simulink model "sampleModel1861"  (R2023a)
settings: Solver=VariableStepAuto  StartTime=0.0  StopTime=10.0  RelTol=1e-3
libraries: simulink x6, hdlsllib x5
settings Model: Creator=user1  LastModifiedBy=user1

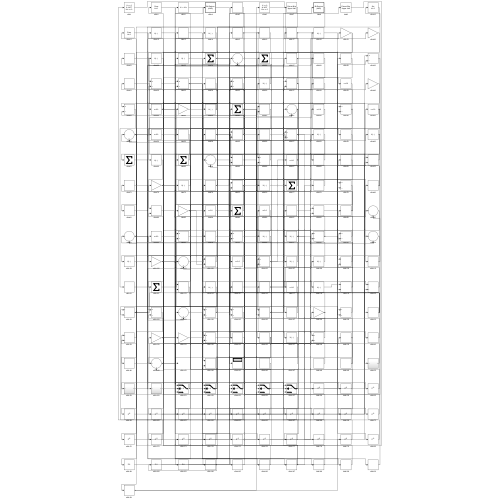
[thumbnail: Simulink's stored preview of the top-level diagram]
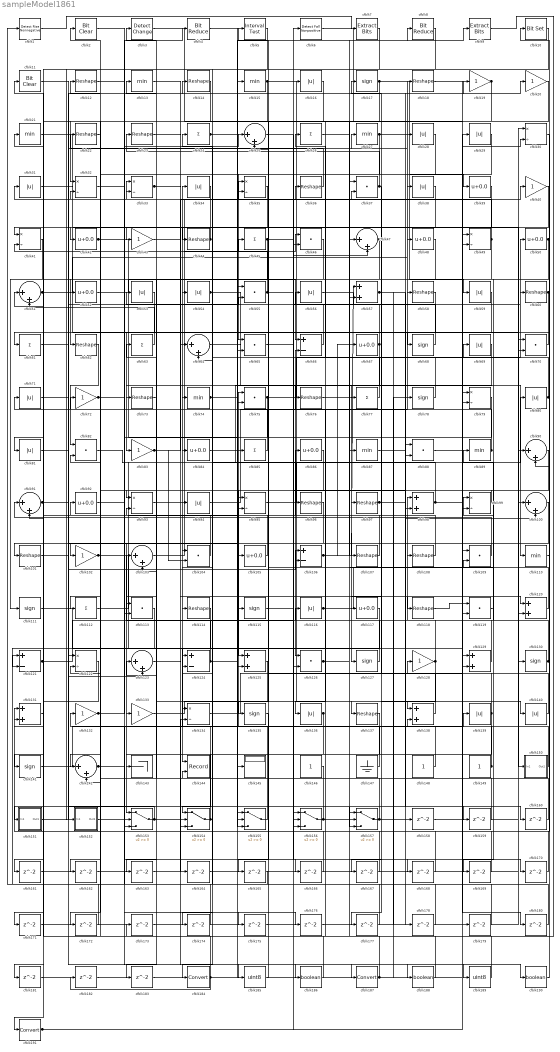
== system sampleModel1861 ==
  cfblk1 : hdlsllib/Logic and Bit Operations/Detect Rise Nonnegative  vinit=0  OutDataTypeStr=boolean
  cfblk10 : simulink/Logic and Bit Operations/Bit Set  iBit=0
      settings: LibrarySourceBlock=|
      | hdlsllib/Logic and Bit
      | Operations/Bit Set
  cfblk{25,47,51,64,90..91,100,103,123,142} (10 alike) : Sum  Inputs=|++
  cfblk{12,14,18,22..23,36,44,58,60,62,73,76,96..97,101,107..108,114,118,137} (20 alike) : Reshape
  cfblk{19..20,40,43,72,83,102,128,132..133} (10 alike) : Gain
  cfblk{37,46,55,65,70,75,82,88,104,109,113,119,126} (13 alike) : DotProduct  OutDataTypeStr=Inherit: Inherit via internal rule
  cfblk{39,42,48,50,52,67,84,86,92,105,117} (11 alike) : Bias  Bias=0.0  SaturateOnIntegerOverflow=off
  cfblk{66,106,121,124} (4 alike) : Sum  Inputs=+-
  cfblk11 : simulink/Logic and Bit Operations/Bit Clear  iBit=0
      settings: LibrarySourceBlock=|
      | hdlsllib/Logic and Bit
      | Operations/Bit Clear
  cfblk{13,15,21,27,74,87,89,110} (8 alike) : MinMax
  cfblk{17,68,78,111,115,127,130,135,141} (9 alike) : Signum
  cfblk{24,26,45,61,63,77,85,112} (8 alike) : Sum  Inputs=+
  cfblk{16,28..29,31,34,38,53..54,56,59,69,71,80..81,94,116,136,139..140} (19 alike) : Abs  SaturateOnIntegerOverflow=off
  cfblk{57,98,120,125,129,131,138} (7 alike) : Sum
  cfblk{30,32..33,35,41,49,79,93,95,99,122,134} (12 alike) : Product  Inputs=*/  RndMeth=Zero  SaturateOnIntegerOverflow=on
  cfblk143 : Terminator
  cfblk144 : Record  FileSettingsInternal="{\"entries\":[{\"content\":{\"excelSettings\":{\"content\":{},\"type\":\"Streamout.ExcelSettings\"}},\"type\":\"Streamout.FileSettingStorage\",\"uuid\":\"\"}],\"packageUris\":[\"http:\\/\\/schema.mathworks.com\\/mf0\\/streamout_blocks\\/R2020a\"],\"version\":\"1.0\"}"  Layout=[1 1]  SignalsInternal="{\"entries\":[{\"content\":{\"signals\":[{\"content\":{\"blockPath\":[],\"dimensions\":[1],\"domain\":\"\",\"lineColor\":\"#a2142f\",\"plots\":[1],\"port\":1,\"signalID\":4612,\"signalName\":\"XY Graph:1\"},\"type\":\"RecordBlkView.Signal\",\"uuid\":\"\"},{\"content\":{\"blockPath\":[],\"dimensions\":[1],\"domain\":\"\",\"lineColor\":\"#139fff\",\"plots\":[1],\"port\":2,\"signalID\":4615,\"signalName\":\"XY Graph:2\"},\"type\":\"RecordBlkView.Signal\",\"uuid\":\"\"}]},\"type\":\"RecordBlkView.InputSignals\",\"uuid\":\"\"}],\"packageUris\":[\"http:\\/\\/schema.mathworks.com\\/mf0\\/streamout_blocks\\/R2020a\"],\"version\":\"1.0\"}"  VisualizationBindings="{\"xyplotplugin\":{\"info\":[{\"series\":[{\"bindingParametersList\":[{\"parameter\":\"X-Axis\",\"signalID\":4612,\"signalName\":\"XY Graph:1\"},{\"parameter\":\"Y-Axis\",\"signalID\":4615,\"signalName\":\"XY Graph:2\"}],\"seriesID\":8507}],\"subplotID\":1}]}}"  CompatibilityTag=XY  st=-1
  cfblk145 : Display
  cfblk146 : Constant  SampleTime=-1
  cfblk147 : Ground
  cfblk148 : Constant  SampleTime=-1
  cfblk149 : Constant  SampleTime=-1
  cfblk150 : Subsystem
      settings: LibrarySourceBlock=|
      | hdlsllib/Ports &
      | Subsystems/Subsystem
  cfblk151 : Subsystem
      settings: LibrarySourceBlock=|
      | hdlsllib/Ports &
      | Subsystems/Subsystem
  cfblk152 : Subsystem
      settings: LibrarySourceBlock=|
      | hdlsllib/Ports &
      | Subsystems/Subsystem
  cfblk{153..157} (5 alike) : Switch  SaturateOnIntegerOverflow=off  InputSameDT=off
  cfblk{158..183} (26 alike) : Delay  SampleTime=1
  cfblk184 : DataTypeConversion  SaturateOnIntegerOverflow=off  RndMeth=Floor
  cfblk185 : DataTypeConversion  OutDataTypeStr=uint8  SaturateOnIntegerOverflow=off  RndMeth=Floor
  cfblk186 : DataTypeConversion  OutDataTypeStr=boolean  SaturateOnIntegerOverflow=off  RndMeth=Floor
  cfblk187 : DataTypeConversion  SaturateOnIntegerOverflow=off  RndMeth=Floor
  cfblk188 : DataTypeConversion  OutDataTypeStr=boolean  SaturateOnIntegerOverflow=off  RndMeth=Floor
  cfblk189 : DataTypeConversion  OutDataTypeStr=uint8  SaturateOnIntegerOverflow=off  RndMeth=Floor
  cfblk190 : DataTypeConversion  OutDataTypeStr=boolean  SaturateOnIntegerOverflow=off  RndMeth=Floor
  cfblk191 : DataTypeConversion  SaturateOnIntegerOverflow=off  RndMeth=Floor
  cfblk2 : simulink/Logic and Bit Operations/Bit Clear  iBit=0
      settings: LibrarySourceBlock=|
      | hdlsllib/Logic and Bit
      | Operations/Bit Clear
  cfblk3 : simulink/Logic and Bit Operations/Detect Change  vinit=0  OutDataTypeStr=boolean
      settings: LibrarySourceBlock=|
      | hdlsllib/Logic and Bit
      | Operations/Detect
      | Change
  cfblk4 : hdlsllib/Logic and Bit Operations/Bit Reduce  mode=AND
  cfblk5 : hdlsllib/Logic and Bit Operations/Interval Test  IntervalClosedRight=on  uplimit=0.5  IntervalClosedLeft=on  lowlimit=-0.5  OutDataTypeStr=boolean
  cfblk6 : hdlsllib/Logic and Bit Operations/Detect Fall Nonpositive  vinit=0  OutDataTypeStr=boolean
  cfblk7 : simulink/Logic and Bit Operations/Extract Bits  bitsToExtract=Upper half  numBits=8  bitIdxRange=[0 7]  outScalingMode=Preserve fixed-point scaling
      settings: LibrarySourceBlock=|
      | hdlsllib/Logic and Bit
      | Operations/Extract Bits
  cfblk8 : hdlsllib/Logic and Bit Operations/Bit Reduce  mode=AND
  cfblk9 : simulink/Logic and Bit Operations/Extract Bits  bitsToExtract=Upper half  numBits=8  bitIdxRange=[0 7]  outScalingMode=Preserve fixed-point scaling
      settings: LibrarySourceBlock=|
      | hdlsllib/Logic and Bit
      | Operations/Extract Bits
  wires:
  cfblk108/1 -> cfblk75/1
  cfblk155/1 -> cfblk132/1
  cfblk150/1(Out1) -> cfblk75/2
  cfblk53/1 -> cfblk83/1
  cfblk82/1 -> cfblk110/1
  cfblk8/1 -> cfblk152/1(In1)
  cfblk96/1 -> cfblk153/1
  cfblk15/1 -> cfblk137/1, cfblk142/2
  cfblk138/1 -> cfblk128/1
  cfblk109/1 -> cfblk91/1
  cfblk118/1 -> cfblk119/1
  cfblk133/1 -> cfblk138/1
  cfblk113/1 -> cfblk133/1
  cfblk52/1 -> cfblk66/1
  cfblk105/1 -> cfblk51/1
  cfblk66/1 -> cfblk56/1
  cfblk86/1 -> cfblk125/1
  cfblk116/1 -> cfblk89/1, cfblk108/1
  cfblk18/1 -> cfblk109/1
  cfblk38/1 -> cfblk101/1
  cfblk75/1 -> cfblk50/1, cfblk153/3
  cfblk125/1 -> cfblk143/1
  cfblk124/1 -> cfblk34/1, cfblk9/1
  cfblk42/1 -> cfblk145/1, cfblk129/2
  cfblk17/1 -> cfblk59/1, cfblk57/2
  cfblk67/1 -> cfblk24/1, cfblk113/1
  cfblk154/1 -> cfblk12/1, cfblk124/2
  cfblk76/1 -> cfblk127/1
  cfblk60/1 -> cfblk61/1, cfblk103/2
  cfblk93/1 -> cfblk46/1
  cfblk72/1 -> cfblk166/1, cfblk188/1
  cfblk156/1 -> cfblk123/1, cfblk8/1
  cfblk149/1 -> cfblk63/1, cfblk96/1
  cfblk78/1 -> cfblk26/1
  cfblk33/1 -> cfblk118/1, cfblk185/1
  cfblk134/1 -> cfblk29/1
  cfblk54/1 -> cfblk126/1, cfblk150/1(In1)
  cfblk48/1 -> cfblk62/1
  cfblk62/1 -> cfblk82/1
  cfblk136/1 -> cfblk154/1, cfblk174/1
  cfblk107/1 -> cfblk86/1
  cfblk73/1 -> cfblk33/1
  cfblk61/1 -> cfblk123/2
  cfblk106/1 -> cfblk57/1, cfblk67/1
  cfblk41/1 -> cfblk111/1
  cfblk89/1 -> cfblk72/1, cfblk13/1
  cfblk30/1 -> cfblk131/1
  cfblk141/1 -> cfblk88/1
  cfblk24/1 -> cfblk125/2, cfblk140/1
  cfblk112/1 -> cfblk80/1
  cfblk94/1 -> cfblk66/2
  cfblk28/1 -> cfblk65/1
  cfblk39/1 -> cfblk102/1
  cfblk98/1 -> cfblk74/1, cfblk180/1
  cfblk64/1 -> cfblk130/1
  cfblk81/1 -> cfblk27/1
  cfblk37/1 -> cfblk23/1, cfblk167/1
  cfblk84/1 -> cfblk18/1
  cfblk103/1 -> cfblk16/1
  cfblk131/1 -> cfblk71/1
  cfblk111/1 -> cfblk126/2
  cfblk10/1 -> cfblk191/1
  cfblk80/1 -> cfblk31/1, cfblk69/1
  cfblk147/1 -> cfblk84/1
  cfblk22/1 -> cfblk112/1
  cfblk49/1 -> cfblk77/1, cfblk156/2, cfblk32/2
  cfblk7/1 -> cfblk44/1
  cfblk87/1 -> cfblk20/1
  cfblk119/1 -> cfblk99/1
  cfblk85/1 -> cfblk21/1
  cfblk27/1 -> cfblk39/1, cfblk124/1
  cfblk130/1 -> cfblk95/1, cfblk98/1, cfblk109/2, cfblk103/1, cfblk93/2
  cfblk122/1 -> cfblk141/1
  cfblk6/1 -> cfblk49/2
  cfblk153/1 -> cfblk151/1(In1), cfblk176/1
  cfblk11/1 -> cfblk187/1
  cfblk46/1 -> cfblk73/1
  cfblk21/1 -> cfblk119/2
  cfblk1/1 -> cfblk7/1
  cfblk47/1 -> cfblk91/2, cfblk154/2
  cfblk151/1(Out1) -> cfblk19/1
  cfblk110/1 -> cfblk90/2
  cfblk128/1 -> cfblk116/1, cfblk177/1
  cfblk68/1 -> cfblk3/1
  cfblk129/1 -> cfblk114/1
  cfblk121/1 -> cfblk6/1, cfblk106/2, cfblk190/1
  cfblk104/1 -> cfblk94/1
  cfblk45/1 -> cfblk120/1, cfblk113/2, cfblk98/2
  cfblk40/1 -> cfblk117/1
  cfblk70/1 -> cfblk68/1
  cfblk114/1 -> cfblk121/2
  cfblk95/1 -> cfblk70/1
  cfblk50/1 -> cfblk65/2, cfblk169/1
  cfblk101/1 -> cfblk28/1
  cfblk91/1 -> cfblk122/1, cfblk154/3
  cfblk77/1 -> cfblk53/1
  cfblk127/1 -> cfblk104/1
  cfblk44/1 -> cfblk43/1, cfblk41/1
  cfblk142/1 -> cfblk139/1, cfblk157/2
  cfblk26/1 -> cfblk107/1
  cfblk71/1 -> cfblk105/1
  cfblk79/1 -> cfblk93/1
  cfblk102/1 -> cfblk144/1, cfblk55/1
  cfblk69/1 -> cfblk134/1
  cfblk157/1 -> cfblk45/1, cfblk129/1
  cfblk43/1 -> cfblk64/1
  cfblk35/1 -> cfblk42/1
  cfblk3/1 -> cfblk79/1
  cfblk57/1 -> cfblk100/2, cfblk178/1
  cfblk146/1 -> cfblk144/2
  cfblk59/1 -> cfblk99/2
  cfblk132/1 -> cfblk14/1, cfblk157/3
  cfblk56/1 -> cfblk58/1
  cfblk148/1 -> cfblk106/1
  cfblk97/1 -> cfblk158/1, cfblk159/1
  cfblk83/1 -> cfblk36/1, cfblk104/2
  cfblk25/1 -> cfblk47/2
  cfblk115/1 -> cfblk60/1
  cfblk99/1 -> cfblk97/1
  cfblk16/1 -> cfblk135/1
  cfblk140/1 -> cfblk17/1
  cfblk152/1(Out1) -> cfblk138/2
  cfblk139/1 -> cfblk85/1, cfblk155/3
  cfblk32/1 -> cfblk4/1
  cfblk74/1 -> cfblk54/1, cfblk37/2
  cfblk14/1 -> cfblk32/1
  cfblk92/1 -> cfblk25/1
  cfblk88/1 -> cfblk30/2
  cfblk126/1 -> cfblk87/1, cfblk38/1
  cfblk36/1 -> cfblk22/1
  cfblk19/1 -> cfblk81/1, cfblk136/1
  cfblk90/1 -> cfblk142/1
  cfblk31/1 -> cfblk100/1
  cfblk5/1 -> cfblk184/1
  cfblk63/1 -> cfblk51/2
  cfblk51/1 -> cfblk48/1, cfblk55/2, cfblk181/1
  cfblk20/1 -> cfblk52/1
  cfblk55/1 -> cfblk40/1, cfblk41/2
  cfblk120/1 -> cfblk35/1
  cfblk158/1 -> cfblk70/2
  cfblk159/1 -> cfblk122/2
  cfblk4/1 -> cfblk160/1
  cfblk160/1 -> cfblk33/2
  cfblk100/1 -> cfblk161/1
  cfblk161/1 -> cfblk30/1
  cfblk29/1 -> cfblk162/1
  cfblk162/1 -> cfblk134/2
  cfblk58/1 -> cfblk163/1
  cfblk163/1 -> cfblk47/1
  cfblk123/1 -> cfblk164/1
  cfblk164/1 -> cfblk90/1
  cfblk135/1 -> cfblk165/1
  cfblk165/1 -> cfblk1/1
  cfblk166/1 -> cfblk35/2
  cfblk167/1 -> cfblk156/1
  cfblk23/1 -> cfblk168/1
  cfblk168/1 -> cfblk25/2
  cfblk169/1 -> cfblk82/2
  cfblk65/1 -> cfblk170/1
  cfblk170/1 -> cfblk49/1
  cfblk117/1 -> cfblk171/1
  cfblk171/1 -> cfblk155/2
  cfblk34/1 -> cfblk172/1
  cfblk172/1 -> cfblk121/1
  cfblk9/1 -> cfblk173/1
  cfblk173/1 -> cfblk120/2
  cfblk174/1 -> cfblk153/2
  cfblk12/1 -> cfblk175/1
  cfblk175/1 -> cfblk46/2
  cfblk176/1 -> cfblk88/2
  cfblk177/1 -> cfblk157/1
  cfblk178/1 -> cfblk64/2
  cfblk179/1 -> cfblk155/1
  cfblk180/1 -> cfblk131/2
  cfblk181/1 -> cfblk79/2
  cfblk182/1 -> cfblk95/2
  cfblk137/1 -> cfblk183/1
  cfblk183/1 -> cfblk15/1
  cfblk184/1 -> cfblk182/1, cfblk92/1
  cfblk185/1 -> cfblk5/1
  cfblk13/1 -> cfblk186/1
  cfblk186/1 -> cfblk11/1
  cfblk187/1 -> cfblk76/1, cfblk37/1, cfblk78/1
  cfblk188/1 -> cfblk2/1
  cfblk2/1 -> cfblk189/1
  cfblk189/1 -> cfblk115/1
  cfblk190/1 -> cfblk10/1
  cfblk191/1 -> cfblk179/1, cfblk156/3

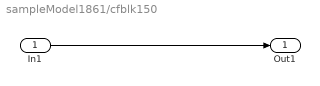
== system sampleModel1861/cfblk150 ==
  In1 : Inport
  Out1 : Outport
  wires:
  In1/1 -> Out1/1

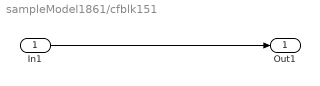
== system sampleModel1861/cfblk151 ==
  In1 : Inport
  Out1 : Outport
  wires:
  In1/1 -> Out1/1

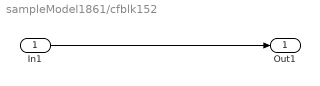
== system sampleModel1861/cfblk152 ==
  In1 : Inport
  Out1 : Outport
  wires:
  In1/1 -> Out1/1
